simulink model "prob3_msd"  (R2024a)
settings: Solver=VariableStepAuto  StartTime=0.0  StopTime=10.0  RelTol=1e-3
settings Model: Creator=yeseo  LastModifiedBy=yeseo

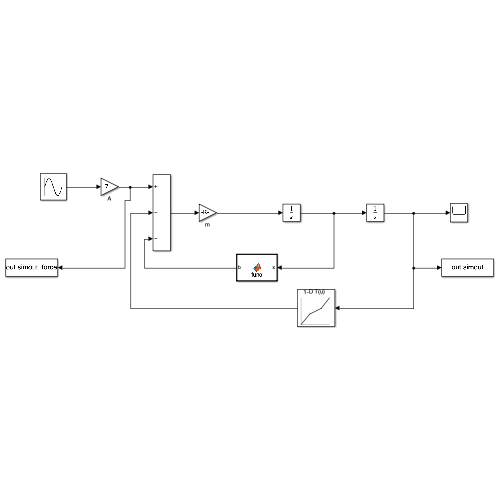
[thumbnail: Simulink's stored preview of the top-level diagram]
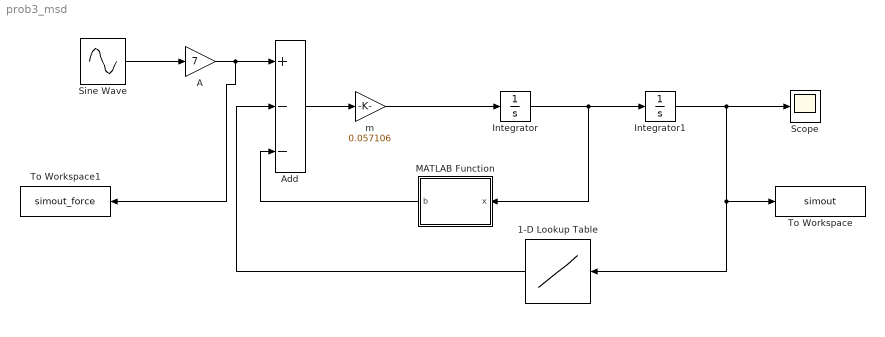
== system prob3_msd ==
  1-D Lookup Table : Lookup_n-D  NumberOfTableDimensions=1  BreakpointsForDimension1=[-10 -4 4 10]  Table=[-5 -1 1 5]  InternalRulePriority=Speed  RndMeth=Simplest
  A : Gain  Gain=7
  Add : Sum  Inputs=+--
  Integrator : Integrator
  Integrator1 : Integrator
  MATLAB Function : MATLAB Function  TreatAsAtomicUnit=on
  Scope : Scope
  Sine Wave : Sin  Frequency=10  SampleTime=0
  To Workspace : ToWorkspace  VariableName=simout  SampleTime=-1
  To Workspace1 : ToWorkspace  VariableName=simout_force  SampleTime=-1
  m : Gain  Gain=0.057106
  wires:
  Sine Wave/1 -> A/1
  Integrator1/1 -> To Workspace/1, 1-D Lookup Table/1, Scope/1
  Integrator/1 -> MATLAB Function/1(x), Integrator1/1
  Add/1 -> m/1
  m/1 -> Integrator/1
  A/1 -> To Workspace1/1, Add/1
  MATLAB Function/1(b) -> Add/3
  1-D Lookup Table/1 -> Add/2

== matlab function prob3_msd/MATLAB Function ==
  data: x input; b output
function b = func(x)

if x>0
    b = 3.5*x.^0.6;
else
    b = -5.5*abs(x).^0.6;
end
